simulink model "boatx010"  (R2019b)
settings: Solver=ode4  StartTime=0.0  StopTime=20  FixedStep=0.01  RelTol=1e-3  EnableMultiTasking=on
values from neighbouring files (symbols this model uses):
  A = 10    [sm_boat_runx010.m]
  a1 = a1n(nx)    [sm_boat_runx010.m]
  a2 = a2n(nx)    [sm_boat_runx010.m]
  a3 = a3n(nx)    [sm_boat_runx010.m]
  aa = 50    [sm_boat_runx010.m]
  B = 10    [sm_boat_runx010.m]
  bmax = pi*(0.47)    (= 1.47654854719)    [sm_boat_runx010.m]
  d1 = d1n(nx)    [sm_boat_runx010.m]
  d2 = d2n(nx)    [sm_boat_runx010.m]
  d3 = d3n(nx)    [sm_boat_runx010.m]
  fixedstep = 0.01    [sm_boat_runx010.m]
  Fmax = 20    [sm_boat_runx010.m]
  H = 0.20    (= 0.2)    [sm_boat_runx010.m]
  Iz = m*(W^2+L^2)/12    (= 0.759791666667)    [sm_boat_runx010.m]
  Izz = (0.1*m*W^2+1000*pi*D^2*L^3)/2/12    (= 0.336072151416)    [sm_boat_runx010.m]
  kai = pi*2/8    (= 0.785398163397)    [sm_boat_runx010.m]
  L = 1    [sm_boat_runx010.m]
  Lt = 0.4    [sm_boat_runx010.m]
  m = 7    [sm_boat_runx010.m]
  mxx = 0.05*m    (= 0.35)    [sm_boat_runx010.m]
  myy = 1000*pi*D^2*L/2    (= 3.92699081699)    [sm_boat_runx010.m]
  n_o_w = length(wps)    [sm_boat_runx010.m]
  td = 0    [sm_boat_runx010.m]
  W = 0.55    [sm_boat_runx010.m]
  wd = fd*2*pi    (= 0.628318530718)    [sm_boat_runx010.m]
  wp_sh = 10    [sm_boat_runx010.m]
  wp_tol = 1    [sm_boat_runx010.m]
  wps = [0 0; -aa -aa; aa -aa; aa/2 -aa/2; aa/2 aa/2; aa aa; -aa aa; -aa/2 aa/2; -aa/2 0; -aa/5 0]    [sm_boat_runx010.m]
undefined symbols (not defined in the file or in its folder): X, Y, Z
libraries: sm_lib x36, nesl_utility x11
(part 2 of 2)

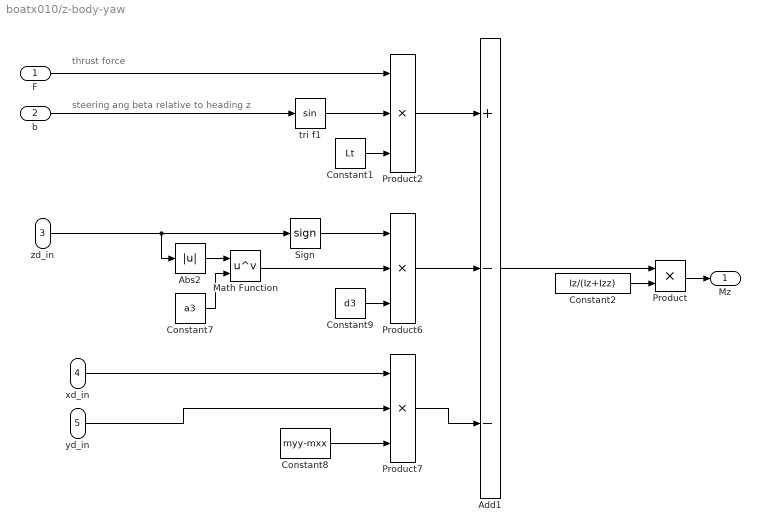
== system boatx010/z-body-yaw ==
  note: thrust force
  note: steering ang beta relative to heading z
  F : Inport
  b : Inport  Port=2
  zd_in : Inport  Port=3
  xd_in : Inport  Port=4
  yd_in : Inport  Port=5
  Abs2 : Abs
  Add1 : Sum  Inputs=+--
  Constant1 : Constant  Value=Lt
  Constant2 : Constant  Value=Iz/(Iz+Izz)
  Constant7 : Constant  Value=a3
  Constant8 : Constant  Value=myy-mxx  VectorParams1D=off
  Constant9 : Constant  Value=d3
  Math Function : Math  Operator=pow  SaturateOnIntegerOverflow=on
  Product : Product
  Product2 : Product  Inputs=3
  Product6 : Product  Inputs=3
  Product7 : Product  Inputs=3
  Sign : Signum
  tri f1 : Trigonometry
  Mz : Outport  VectorParamsAs1DForOutWhenUnconnected=off
  wires:
  F/1 -> Product2/1
  tri f1/1 -> Product2/2
  b/1 -> tri f1/1
  Product2/1 -> Add1/1
  Constant1/1 -> Product2/3
  zd_in/1 -> Sign/1, Abs2/1
  Product7/1 -> Add1/3
  xd_in/1 -> Product7/1
  yd_in/1 -> Product7/2
  Constant8/1 -> Product7/3
  Product6/1 -> Add1/2
  Abs2/1 -> Math Function/1
  Constant7/1 -> Math Function/2
  Math Function/1 -> Product6/2
  Constant9/1 -> Product6/3
  Sign/1 -> Product6/1
  Add1/1 -> Product/1
  Constant2/1 -> Product/2
  Product/1 -> Mz/1

== matlab function boatx010/counter ==
  data: dst input; wp_tol input; wcount output; A data_store_memory
function wcount = checkDistance(dst,wp_tol)
global A
if dst < wp_tol
    A= A+1;
end
   
wcount = A;

== matlab function boatx010/MATLAB Function1 ==
  data: F output; b output; X input; Xw input; Y input; Yw input; z input; Fmax input; bmax input; wp_sh input; hd output; dhd output; dst output; wp_tol input
function [F,b,hd,dhd,dst] = nav(X,Xw,Y,Yw,z,Fmax,bmax,wp_sh,wp_tol)
% #codegen
% Xw Yw - m, current waypoint
% X Y - m, current position
% z - rad, current heading
% V - m/s, forward speed demand
% Fmax - N, max thrust force 
% b - rad, max thruster steer angle demand
% YH 2017-03-25

Xdiff = Xw - X ; % m, X position error
Ydiff = Yw - Y ;
dst = sqrt(Xdiff^2 + Ydiff^2) ; % m, distance to next waypoint
% dst = norm([Xw Yw],[X Y]) ;

hd = atan2(Ydiff,Xdiff) ; % rad, heading demand by calculation
% atan2(y,x) returns 4 quadrant inverse tangent in range [-pi, pi]

% if hd < -pi % negative heading demand too large
%     hd = 2*pi + hd ; % corrected hd    
% elseif hd > pi % positive heading demand too large
%     hd = -2*pi + hd ; % corrected hd
% end

if z < -pi % negative current heading too large
    z = 2*pi + z ; % corrected current heading    
elseif z > pi % positive current heading too large
    z = -2*pi + z ; % corrected
end

dhd = hd - z ; % rad, different between demand and current heading

if dhd < -pi % negative heading difference too large
    dhd = 2*pi + dhd ; % corrected dhd    
elseif dhd > pi % positive heading difference too large
    dhd = -2*pi + dhd ; % corrected
end

F = 0 ;
b = 0 ;

if (dhd > -pi/2) && (dhd < pi/2) % heading difference small        
    b = bmax*dhd/(pi/2) ; % thruster angle proportional to heading difference
    F = Fmax ;
elseif ((dhd >= -pi)&&(dhd <= -pi/2)) || ((dhd >= pi/2)&&(dhd <= pi)) % heading difference large
    b = bmax*(sign(dhd)) ; % thruster angle maximum
    if (dst <= wp_sh) % remaining distance too short for turn at large heading difference 
        F = (Fmax/3)*(dst/wp_sh) ; % thrust proportional to distance and limited to a third of max
    else
        F = Fmax/2 ; % thrust limited to half max
    end
end

end


%{
if dhd < -pi % negative heading difference too large
    dhd = 2*pi + hd - z ; % add 2*pi to avoid swirl
    hd = 2*pi + hd ; % to display the corrected hd
elseif dhd > pi % positive heading difference too large
    dhd = -2*pi + hd - z ; % add -2*pi to avoid swirl
    hd = -2*pi + hd ; % corrected hd
end

if (dst <= wp_tol) % close to waypoint
    F = 0 ; % stop engine
    b = 0 ;
else
    if (dhd > -pi/2) && (dhd < pi/2) % heading difference small
%         b = bmax*dhd/(pi/2) ; % thruster angle proportional to heading difference
        b = bmax*dhd/(pi/2) ; % thruster angle proportional to heading difference
        F = Fmax ;
    elseif ((dhd >= -pi)&&(dhd <= -pi/2)) || ((dhd >= pi/2)&&(dhd <= pi)) % heading difference large
        b = bmax*(sign(dhd)) ; % thruster angle maximum
        if (dst <= wp_sh) % remaining distance too short for turn at large heading difference 
            F = (Fmax/3)*(dst/wp_sh) ; % thrust proportional to distance and limited to a third of max
        else
            F = Fmax/2 ; % thrust limited to half max
        end
    end
end
%}


% if (Xdiff>0)&&(Ydiff>0) % 1st quadrant
%     hd_rad = atan(Ydiff/Xdiff) ;
% elseif (Xdiff>0)&&(Ydiff<0) % 4th quadrant
%     hd_rad = atan(Ydiff/Xdiff) ;
% elseif (Xdiff<0)&&(Ydiff>0) % 2nd quadrant 
%     hd_rad = pi + atan(Ydiff/Xdiff) ;
% elseif (Xdiff<0)&&(Ydiff<0) % 3rd quadrant
%     hd_rad = -pi + atan(Ydiff/Xdiff) ;
% end

% if (Xdiff>0.01) && (Ydiff>0.01) % 1st quadrant
%     hd_rad = atan(Ydiff/Xdiff) ;
% elseif (Xdiff>0.01) && (Ydiff<-0.01) % 4th quadrant
%     hd_rad = atan(Ydiff/Xdiff) ;
% elseif (Xdiff<-0.01) && (Ydiff>0.01) % 2nd quadrant 
%     hd_rad = pi + atan(Ydiff/Xdiff) ;
% elseif (Xdiff<-0.01) && (Ydiff<-0.01) % 3rd quadrant
%     hd_rad = -pi + atan(Ydiff/Xdiff) ;
% elseif (-0.01<=Xdiff<=0.01) && (Ydiff>=0.01) % when reaching Xw not Yw
%     hd_rad = pi/2 ; 
% elseif (-0.01<=Xdiff<=0.01) && (Ydiff<=-0.01)
%     hd_rad = -pi/2 ;
% elseif (Xdiff>=0.01) && (-0.01<=Ydiff<=0.01) % when reaching Yw not Xw
%     hd_rad = 0 ;
% elseif (Xdiff<=-0.01) && (-0.01<=Ydiff<=0.01)
%     hd_rad = pi ;
% end

== matlab function boatx010/STOP/MATLAB Function ==
  data: arrayLength input; Wp input; io output; dst input; wp_tol input
function io  = shutoff(arrayLength,Wp,dst,wp_tol)
%#codegen

io = 0;

if [(dst <= wp_tol) && (Wp == arrayLength)]
    io = 1;
else
    io = 0;
end
end
